simulink model "clik_inverse"  (R2022b)
settings: Solver=ode1  StartTime=0.0  StopTime=4  FixedStep=0.001  RelTol=1e-3
undefined symbols (not defined in the file or in its folder): DiscIntNeverNeededParam, q0, Tc
settings Model: Creator=Xp  LastModifiedBy=brigh
settings SolverCC: AlgebraicLoopSolver=TrustRegion
settings DataIOCC: LimitDataPoints=on  SaveFormat=Array  SignalLoggingSaveFormat=ModelDataLogs  ReturnWorkspaceOutputs=off
settings OptimizationCC: ExpressionDepthLimit=2147483647  InitFltsAndDblsToZero=on  LifeSpan=inf
settings DebuggingCC: SaveWithParameterizedLinksMsg=none  UnderspecifiedInitializationDetection=Classic  MergeDetectMultiDrivingBlocksExec=none  SolverPrmCheckMsg=warning  MultiTaskDSMMsg=warning  MultiTaskCondExecSysMsg=none  FcnCallInpInsideContextMsg=warning  UnconnectedInputMsg=warning  UnconnectedOutputMsg=warning  UnconnectedLineMsg=warning  StateNameClashWarn=warning  SFUnexpectedBacktrackingDiag=warning  SFNoUnconditionalDefaultTransitionDiag=warning  SFExecutionAtInitializationDiag=none  SFMachineParentedDataDiag=warning  ArithmeticOperatorsInVariantConditions=warning
settings HardwareCC: ProdBitPerPointer=32  ProdBitPerSizeT=32  ProdBitPerPtrDiffT=32  ProdLargestAtomicFloat=None  ProdIntDivRoundTo=Undefined  ProdEndianess=Unspecified  ProdWordSize=32  ProdHWDeviceType=32-bit Generic
settings ModelReferenceCC: EnableRefExpFcnMdlSchedulingChecks=on  PropagateSignalLabelsOutOfModel=off
settings SFSimCC: CustomCodeUndefinedFunction=UseInterfaceOnly
settings RTWCC: DLArmComputeVersion=19.05
settings CodeAppCC: StateflowObjectComments=on
settings GRTTargetCC: TargetLangStandard=C89/C90 (ANSI)  CombineOutputUpdateFcns=off  GRTInterface=on
settings ConfigComp: CovMetricSettings=dw  CovSaveCumulativeToWorkspaceVar=on  CovSaveSingleToWorkspaceVar=on

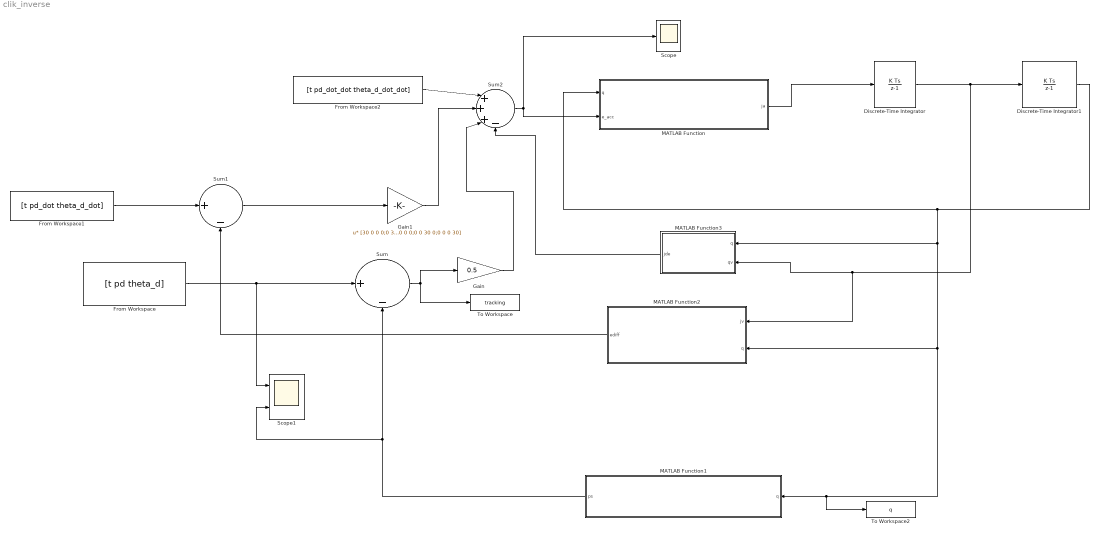
== system clik_inverse ==
  Discrete-Time Integrator : DiscreteIntegrator  SampleTime=Tc  ICPrevOutput=DiscIntNeverNeededParam  ICPrevScaledInput=DiscIntNeverNeededParam
  Discrete-Time Integrator1 : DiscreteIntegrator  InitialCondition=q0  SampleTime=Tc  LimitOutput=on  UpperSaturationLimit=[pi/2; pi/4; 1; 2*pi]  LowerSaturationLimit=[-pi/2; -pi/2; 0.25; -2*pi]  ICPrevOutput=DiscIntNeverNeededParam  ICPrevScaledInput=DiscIntNeverNeededParam
  From Workspace : FromWorkspace  VariableName=[t pd theta_d]  SampleTime=Tc
  From Workspace1 : FromWorkspace  VariableName=[t pd_dot theta_d_dot]  SampleTime=Tc
  From Workspace2 : FromWorkspace  VariableName=[t pd_dot_dot theta_d_dot_dot]  SampleTime=Tc
  Gain : Gain  Gain=0.5
  Gain1 : Gain  Gain=[30 0 0 0;0 30 0 0;0 0 30 0;0 0 0 30]  Multiplication=Matrix(u*K)
  MATLAB Function : MATLAB Function  TreatAsAtomicUnit=on
  MATLAB Function1 : MATLAB Function  TreatAsAtomicUnit=on
  MATLAB Function2 : MATLAB Function  TreatAsAtomicUnit=on
  MATLAB Function3 : MATLAB Function  TreatAsAtomicUnit=on
  Scope : Scope
  Scope1 : Scope  NumInputPorts=2
  Sum : Sum  Inputs=|+-
  Sum1 : Sum  Inputs=|+-
  Sum2 : Sum  Inputs=|+++-
  To Workspace : ToWorkspace  VariableName=tracking  SampleTime=-1
  To Workspace2 : ToWorkspace  VariableName=q  SampleTime=-1
  wires:
  MATLAB Function/1(ja) -> Discrete-Time Integrator/1
  Discrete-Time Integrator/1 -> Discrete-Time Integrator1/1, MATLAB Function2/1(jv), MATLAB Function3/2(qv)
  Discrete-Time Integrator1/1 -> MATLAB Function/1(q), MATLAB Function2/2(q), To Workspace2/1, MATLAB Function1/1(q), MATLAB Function3/1(q)
  MATLAB Function1/1(ps) -> Sum/2, Scope1/2
  From Workspace/1 -> Sum/1, Scope1/1
  Sum/1 -> To Workspace/1, Gain/1
  From Workspace1/1 -> Sum1/1
  Sum1/1 -> Gain1/1
  From Workspace2/1 -> Sum2/1
  Gain1/1 -> Sum2/2
  Gain/1 -> Sum2/3
  MATLAB Function3/1(jde) -> Sum2/4
  Sum2/1 -> Scope/1, MATLAB Function/2(e_acc)
  MATLAB Function2/1(ediff) -> Sum1/2

== matlab function clik_inverse/MATLAB Function1 ==
  data: q input; ps output
function ps = fcn(q)


cos1 = cos(q(1));

cos12 = cos(q(1) + q(2));

cos124 = cos(q(1) + q(2) + q(4));

sin1 = sin(q(1));

sin12 = sin(q(1) + q(2));

sin124 = sin(q(1) + q(2) + q(4));

d3=q(3);


M = [cos124, -sin124, 0, cos12/2 + cos1/2
      sin124, cos124, 0, sin12/2 + sin1/2
       0, 0, 1, 1 - d3
       0, 0, 0, 1];



     

    err = M(1:3,4);
    err = err';
    O = q(1) + q(2) + q(4);
    ps = [err O];


    
end

== matlab function clik_inverse/MATLAB Function ==
  data: q input; ja output; e_acc input
function ja = jacob_inv(q,e_acc)



a1 = 0.5;
a2 = 0.5;
d3 = q(3);

theta1 = q(1);
theta12 = theta1+q(2);

cos1 = cos(theta1);
sin1 = sin(theta1);
cos12 = cos(theta12);
sin12 = sin(theta12);


J = [-a2*sin12-a1*sin1 -a2*sin12 0 0; a2*cos12+a1*cos1 a2*cos12 0 0;0 0 1 0; 1 1 0 1];

    
    jacinv = double(inv(J));
    %xvel = transpose(xvel)
    ja = jacinv*e_acc';

end

== matlab function clik_inverse/MATLAB Function2 ==
  data: jv input; q input; ediff output
function ediff = fcn(jv,q)

a1 = 0.5;
a2 = 0.5;
d3 = q(3);

theta1 = q(1);
theta12 = theta1+q(2);

cos1 = cos(theta1);
sin1 = sin(theta1);
cos12 = cos(theta12);
sin12 = sin(theta12);


J = [-a2*sin12-a1*sin1 -a2*sin12 0 0; a2*cos12+a1*cos1 a2*cos12 0 0;0 0 1 0; 1 1 0 1];



ediff = transpose(J*jv);


end

== matlab function clik_inverse/MATLAB Function3 ==
  data: q input; jde output; qv input
function jde = jacob_diff(q,qv)
    a1 = 0.5;
    a2 = 0.5;
    
    difftheta1 = qv(1);
    difftheta2 = qv(2);
    diffd3 = qv(3);
    difftheta4 = qv(4);

    theta1 = q(1);
    theta2 = q(2);
    d3 = q(3);
    theta4 = q(4);



diffJ = [ -(cos(theta1)*difftheta1)/2 - (cos(theta1 + theta2)*(difftheta1 + difftheta2))/2, -(cos(theta1 + theta2)*(difftheta1 + difftheta2))/2, 0, 0; -(sin(theta1)*difftheta1)/2 - (sin(theta1 + theta2)*(difftheta1 + difftheta2))/2, -(sin(theta1 + theta2)*(difftheta1 + difftheta2))/2, 0, 0; 0, 0, 0, 0;0, 0, 0, 0];

jde = transpose(diffJ*qv);


end
